simulink model "fft_filters"  (R2019b)
settings: Solver=FixedStepDiscrete  StartTime=0.0  StopTime=0.01  RelTol=1e-3
InitFcn:
  | initCallback
StopFcn:
  | stopCallback
undefined symbols (not defined in the file or in its folder): config, mp
libraries: hdlsllib x32, simulink x12, dsphdlxfrm x4, dspsigops x2
(part 1 of 2)
settings Model: DataTypeOverride=Off  SimulationMode=accelerator  Creator=Ross  LastModifiedBy=wickh
settings DataIOCC: ReturnWorkspaceOutputs=off
settings OptimizationCC: BlockReduction=off  ConditionallyExecuteInputs=off  DefaultParameterBehavior=Inlined
settings DebuggingCC: ReadBeforeWriteMsg=DisableAll  WriteAfterWriteMsg=DisableAll  WriteAfterReadMsg=DisableAll  AlgebraicLoopMsg=error  MultiTaskDSMMsg=none  SingleTaskRateTransMsg=error  PregeneratedLibrarySubsystemCodeDiagnostic=none  ArithmeticOperatorsInVariantConditions=warning
settings HardwareCC: ProdBitPerPointer=32  ProdBitPerSizeT=32  ProdBitPerPtrDiffT=32  ProdLargestAtomicFloat=None  ProdIntDivRoundTo=Undefined  ProdEndianess=Unspecified  ProdWordSize=32  ProdHWDeviceType=ASIC/FPGA->ASIC/FPGA  TargetBitPerPointer=64  TargetBitPerSizeT=64  TargetBitPerPtrDiffT=64  TargetLongLongMode=on  TargetIntDivRoundTo=Zero  TargetEndianess=LittleEndian  TargetWordSize=64  TargetHWDeviceType=Custom Processor->MATLAB Host Computer  ProdEqTarget=off
settings ModelReferenceCC: UpdateModelReferenceTargets=IfOutOfDate
settings SFSimCC: SFSimEcho=off  SimUseLocalCustomCode=off  CustomCodeUndefinedFunction=UseInterfaceOnly
settings RTWCC: RTWUseLocalCustomCode=off

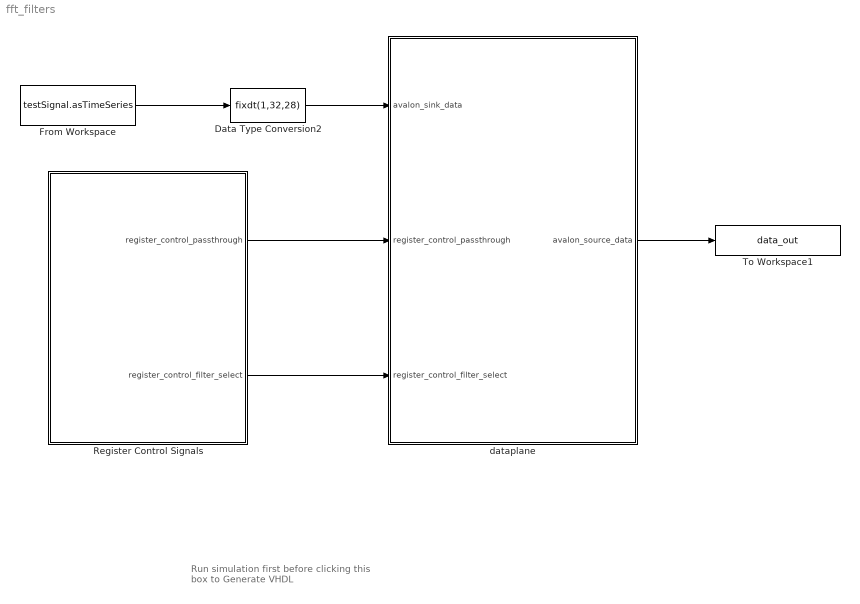
== system fft_filters ==
  note: Run simulation first
      | before clicking this box to
      | Generate VHDL
  Data Type Conversion2 : DataTypeConversion  OutDataTypeStr=fixdt(1,32,28)
  From Workspace : FromWorkspace  VariableName=testSignal.asTimeSeries  SampleTime=1 / config.system.sampleClockFrequency
  Register Control Signals : Subsystem
  To Workspace1 : ToWorkspace  VariableName=data_out  SaveFormat=Timeseries  SampleTime=-1
  dataplane : Subsystem  TreatAsAtomicUnit=on
  wires:
  dataplane/1("avalon_source_data ") -> To Workspace1/1
  Register Control Signals/1(register_control_passthrough) -> dataplane/2(register_control_passthrough)
  Register Control Signals/2(register_control_filter_select) -> dataplane/3(register_control_filter_select)
  From Workspace/1 -> Data Type Conversion2/1
  Data Type Conversion2/1 -> dataplane/1(avalon_sink_data)

== system fft_filters/Register Control Signals ==
  Data Type Conversion1 : DataTypeConversion  OutDataTypeStr=mp.register{2}.dataType  RndMeth=Nearest
  Data Type Conversion2 : DataTypeConversion  OutDataTypeStr=mp.register{1}.dataType  RndMeth=Nearest
  Time Series Signal from Workspace 1 : FromWorkspace  VariableName=mp.register{1}.timeseries  OutDataTypeStr=double  SampleTime=mp.Ts  OutputAfterFinalValue=Holding final value
  Time Series Signal from Workspace 2 : FromWorkspace  VariableName=mp.register{2}.timeseries  OutDataTypeStr=double  SampleTime=mp.Ts  OutputAfterFinalValue=Holding final value
  register_control_passthrough : Outport  VectorParamsAs1DForOutWhenUnconnected=off
  register_control_filter_select : Outport  Port=2  VectorParamsAs1DForOutWhenUnconnected=off
  wires:
  Time Series Signal from Workspace 1/1 -> Data Type Conversion2/1
  Time Series Signal from Workspace 2/1 -> Data Type Conversion1/1
  Data Type Conversion2/1 -> register_control_passthrough/1
  Data Type Conversion1/1 -> register_control_filter_select/1

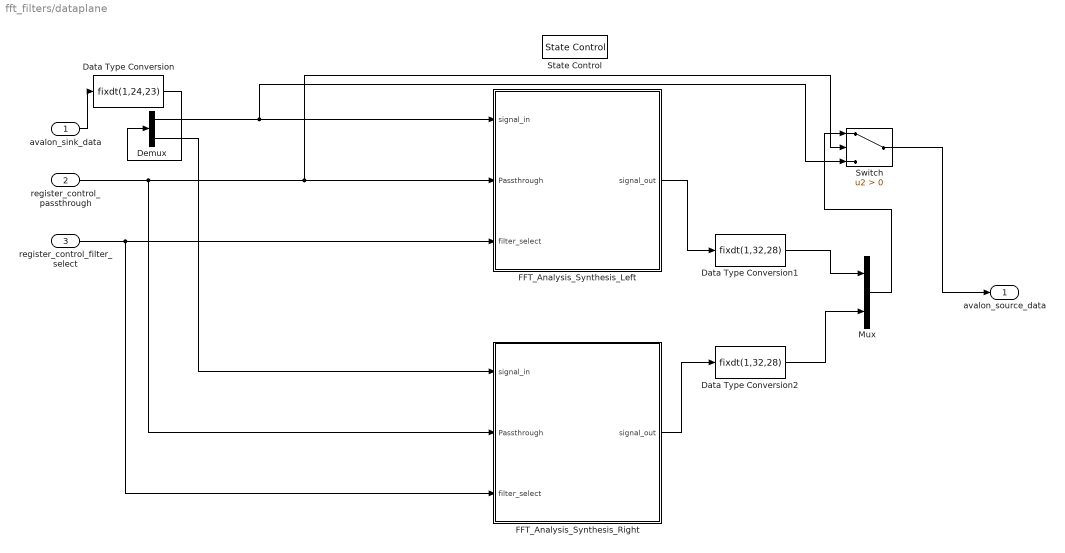
== system fft_filters/dataplane ==
  avalon_sink_data : Inport
  register_control_passthrough : Inport  Port=2
  register_control_filter_select : Inport  Port=3
  Data Type Conversion : DataTypeConversion  OutDataTypeStr=fixdt(1,24,23)
  Data Type Conversion1 : DataTypeConversion  OutDataTypeStr=fixdt(1,32,28)
  Data Type Conversion2 : DataTypeConversion  OutDataTypeStr=fixdt(1,32,28)
  Demux : Demux  Outputs=2
  FFT_Analysis_Synthesis_Left : Subsystem  TreatAsAtomicUnit=on
  FFT_Analysis_Synthesis_Right : Subsystem  TreatAsAtomicUnit=on
  Mux : Mux  Inputs=2
  State Control : StateControl  StateControl=Synchronous
  Switch : Switch  Criteria=u2 > Threshold
  "avalon_source_data " : Outport  InitialOutput=0  VectorParamsAs1DForOutWhenUnconnected=off
  wires:
  Demux/2 -> FFT_Analysis_Synthesis_Right/1(signal_in)
  FFT_Analysis_Synthesis_Right/1(signal_out) -> Data Type Conversion2/1
  avalon_sink_data/1 -> Data Type Conversion/1
  Demux/1 -> Switch/3, FFT_Analysis_Synthesis_Left/1(signal_in)
  FFT_Analysis_Synthesis_Left/1(signal_out) -> Data Type Conversion1/1
  register_control_passthrough/1 -> FFT_Analysis_Synthesis_Right/2(Passthrough), Switch/2, FFT_Analysis_Synthesis_Left/2(Passthrough)
  register_control_filter_select/1 -> FFT_Analysis_Synthesis_Left/3(filter_select), FFT_Analysis_Synthesis_Right/3(filter_select)
  Data Type Conversion/1 -> Demux/1
  Mux/1 -> Switch/1
  Data Type Conversion1/1 -> Mux/1
  Data Type Conversion2/1 -> Mux/2
  Switch/1 -> "avalon_source_data "/1

== system fft_filters/dataplane/FFT_Analysis_Synthesis_Left ==
  note: Gain to normalize
      | sinusoid amplitudes
  signal_in : Inport
  Passthrough : Inport  Port=2
  filter_select : Inport  Port=3
  Analysis : Subsystem
  Frequency_Domain_Processing : Subsystem
  Gain : Gain  OutDataTypeStr=Inherit: Same as input  ParamDataTypeStr=Inherit: Same as input
  Synthesis : Subsystem
  signal_out : Outport  VectorParamsAs1DForOutWhenUnconnected=off
  wires:
  signal_in/1 -> Analysis/1(Signal_in)
  Synthesis/1(synthesized_signal) -> Gain/1
  Analysis/1(FFT_data) -> Frequency_Domain_Processing/1(FFT_results)
  Analysis/2(FFT_valid) -> Frequency_Domain_Processing/2(valid_in)
  Analysis/3(FFT_frame_pulse) -> Frequency_Domain_Processing/3(frame_pulse_in)
  Frequency_Domain_Processing/1(modified_frequencies) -> Synthesis/1(modified_FFT_data)
  Frequency_Domain_Processing/2(valid_out) -> Synthesis/2(FFT_valid)
  Frequency_Domain_Processing/3(frame_pulse_out) -> Synthesis/3(FFT_frame_pulse)
  Analysis/4(passthrough) -> Frequency_Domain_Processing/4(passthrough)
  Passthrough/1 -> Analysis/2(Passthrough)
  Analysis/5(filter_select_out) -> Frequency_Domain_Processing/5(filter_select)
  filter_select/1 -> Analysis/3(filter_select)
  Gain/1 -> signal_out/1

== system fft_filters/dataplane/FFT_Analysis_Synthesis_Right ==
  note: Gain to normalize
      | sinusoid amplitudes
  signal_in : Inport
  Passthrough : Inport  Port=2
  filter_select : Inport  Port=3
  Analysis : Subsystem
  Frequency_Domain_Processing : Subsystem
  Gain : Gain  OutDataTypeStr=Inherit: Same as input  ParamDataTypeStr=Inherit: Same as input
  Synthesis : Subsystem
  signal_out : Outport  VectorParamsAs1DForOutWhenUnconnected=off
  wires:
  signal_in/1 -> Analysis/1(Signal_in)
  Synthesis/1(synthesized_signal) -> Gain/1
  Analysis/1(FFT_data) -> Frequency_Domain_Processing/1(FFT_results)
  Analysis/2(FFT_valid) -> Frequency_Domain_Processing/2(valid_in)
  Analysis/3(FFT_frame_pulse) -> Frequency_Domain_Processing/3(frame_pulse_in)
  Frequency_Domain_Processing/1(modified_frequencies) -> Synthesis/1(modified_FFT_data)
  Frequency_Domain_Processing/2(valid_out) -> Synthesis/2(FFT_valid)
  Frequency_Domain_Processing/3(frame_pulse_out) -> Synthesis/3(FFT_frame_pulse)
  Analysis/4(passthrough) -> Frequency_Domain_Processing/4(passthrough)
  Passthrough/1 -> Analysis/2(Passthrough)
  Analysis/5(filter_select_out) -> Frequency_Domain_Processing/5(filter_select)
  filter_select/1 -> Analysis/3(filter_select)
  Gain/1 -> signal_out/1

== system fft_filters/dataplane/FFT_Analysis_Synthesis_Left/Analysis ==
  note: The ready signal is ignored by design
      | since data won't be sent while FFT
      | engine is busy.
  Signal_in : Inport
  Passthrough : Inport  Port=2
  filter_select : Inport  Port=3
  FFT : dsphdlxfrm/FFT HDL Optimized  FFTLength=mp.FFT_size  Architecture=Burst Radix 2  ComplexMultiplication=Use 4 multipliers and 2 adders  BitReversedOutput=off  BitReversedInput=off  Normalize=off  SimulateUsing=Code generation  RoundingMethod=Floor  ResetInputPort=off  StartOutputPort=off  EndOutputPort=off
      settings: SourceProductName=DSP System Toolbox  SourceProductBaseCode=DS
  FFT Frame Buffering : Subsystem
  Terminator6 : Terminator
  FFT_data : Outport  VectorParamsAs1DForOutWhenUnconnected=off
  FFT_valid : Outport  Port=2  VectorParamsAs1DForOutWhenUnconnected=off
  FFT_frame_pulse : Outport  Port=3  VectorParamsAs1DForOutWhenUnconnected=off
  passthrough : Outport  Port=4
  filter_select_out : Outport  Port=5
  wires:
  FFT/3 -> Terminator6/1
  FFT Frame Buffering/3(FFT_Frame_Start_Pulse) -> FFT_frame_pulse/1
  Signal_in/1 -> FFT Frame Buffering/1(Sample_Data_in)
  FFT Frame Buffering/2(Valid_to_FFT) -> FFT/2
  FFT Frame Buffering/1(Data_to_FFT) -> FFT/1
  FFT/1 -> FFT_data/1
  FFT/2 -> FFT_valid/1
  FFT Frame Buffering/4(passthrough) -> passthrough/1
  Passthrough/1 -> FFT Frame Buffering/2(passthrough_in)
  filter_select/1 -> FFT Frame Buffering/3(filter_select)
  FFT Frame Buffering/5(filter_select_out) -> filter_select_out/1

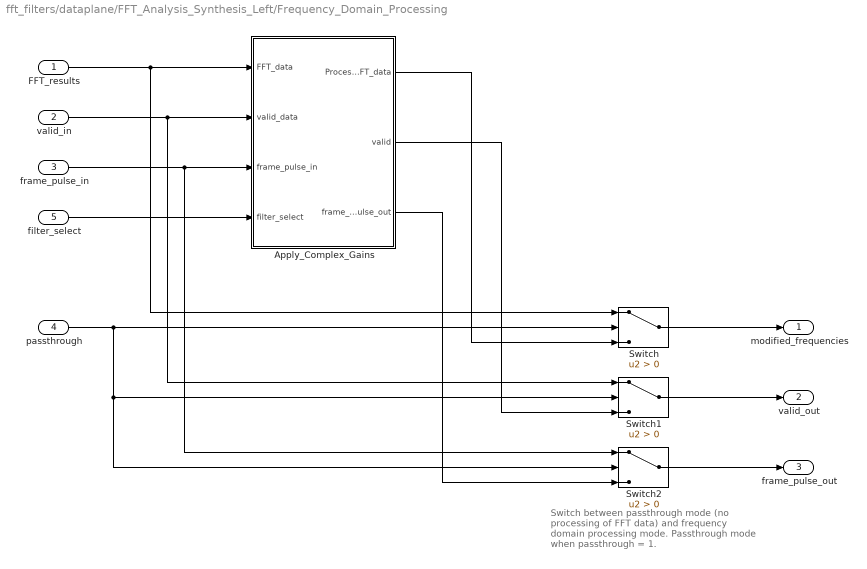
== system fft_filters/dataplane/FFT_Analysis_Synthesis_Left/Frequency_Domain_Processing ==
  note: Switch between passthrough mode
      | (no processing of FFT data)
      | and frequency domain processing mode.
      | Passthrough mode when passthrough = 1.
  FFT_results : Inport
  valid_in : Inport  Port=2
  frame_pulse_in : Inport  Port=3
  passthrough : Inport  Port=4
  filter_select : Inport  Port=5
  Apply_Complex_Gains : Subsystem
  Switch : Switch  Criteria=u2 > Threshold
  Switch1 : Switch  Criteria=u2 > Threshold
  Switch2 : Switch  Criteria=u2 > Threshold
  modified_frequencies : Outport  VectorParamsAs1DForOutWhenUnconnected=off
  valid_out : Outport  Port=2  VectorParamsAs1DForOutWhenUnconnected=off
  frame_pulse_out : Outport  Port=3
  wires:
  FFT_results/1 -> Apply_Complex_Gains/1(FFT_data), Switch/1
  valid_in/1 -> Apply_Complex_Gains/2(valid_data), Switch1/1
  Apply_Complex_Gains/1(Processed_FFT_data) -> Switch/3
  Apply_Complex_Gains/2(valid) -> Switch1/3
  frame_pulse_in/1 -> Apply_Complex_Gains/3(frame_pulse_in), Switch2/1
  passthrough/1 -> Switch2/2, Switch1/2, Switch/2
  Switch/1 -> modified_frequencies/1
  Apply_Complex_Gains/3(frame_pulse_out) -> Switch2/3
  Switch1/1 -> valid_out/1
  Switch2/1 -> frame_pulse_out/1
  filter_select/1 -> Apply_Complex_Gains/4(filter_select)

== system fft_filters/dataplane/FFT_Analysis_Synthesis_Left/Synthesis ==
  note: Making the assumption here
      | that the frequency domain processing
      | preserved the complex conjugate pairs
      | so that the output is real.
  modified_FFT_data : Inport
  FFT_valid : Inport  Port=2
  FFT_frame_pulse : Inport  Port=3
  Data Type Conversion1 : DataTypeConversion  OutDataTypeStr=fixdt(1,mp.W_bits,mp.F_bits)
  Get_Real : ComplexToRealImag
  Overlap_and_Add : Subsystem
  Terminator8 : Terminator
  Terminator9 : Terminator
  iFFT : dsphdlxfrm/IFFT HDL Optimized  FFTLength=mp.FFT_size  Architecture=Burst Radix 2  ComplexMultiplication=Use 4 multipliers and 2 adders  BitReversedOutput=off  BitReversedInput=off  Normalize=on  SimulateUsing=Code generation  RoundingMethod=Floor  ResetInputPort=off  StartOutputPort=off  EndOutputPort=off
      settings: SourceProductName=DSP System Toolbox  SourceProductBaseCode=DS
  synthesized_signal : Outport  VectorParamsAs1DForOutWhenUnconnected=off
  wires:
  iFFT/3 -> Terminator8/1
  iFFT/2 -> Overlap_and_Add/2(iFFT_Valid)
  Get_Real/1 -> Overlap_and_Add/1(IFFT_Data)
  modified_FFT_data/1 -> iFFT/1
  Data Type Conversion1/1 -> synthesized_signal/1
  iFFT/1 -> Get_Real/1
  Get_Real/2 -> Terminator9/1
  FFT_valid/1 -> iFFT/2
  FFT_frame_pulse/1 -> Overlap_and_Add/3(FFT_Frame_Pulse)
  Overlap_and_Add/1(signal_out) -> Data Type Conversion1/1

== system fft_filters/dataplane/FFT_Analysis_Synthesis_Right/Analysis ==
  note: The ready signal is ignored by design
      | since data won't be sent while FFT
      | engine is busy.
  Signal_in : Inport
  Passthrough : Inport  Port=2
  filter_select : Inport  Port=3
  FFT : dsphdlxfrm/FFT HDL Optimized  FFTLength=mp.FFT_size  Architecture=Burst Radix 2  ComplexMultiplication=Use 4 multipliers and 2 adders  BitReversedOutput=off  BitReversedInput=off  Normalize=off  SimulateUsing=Code generation  RoundingMethod=Floor  ResetInputPort=off  StartOutputPort=off  EndOutputPort=off
      settings: SourceProductName=DSP System Toolbox  SourceProductBaseCode=DS
  FFT Frame Buffering : Subsystem
  Terminator6 : Terminator
  FFT_data : Outport  VectorParamsAs1DForOutWhenUnconnected=off
  FFT_valid : Outport  Port=2  VectorParamsAs1DForOutWhenUnconnected=off
  FFT_frame_pulse : Outport  Port=3  VectorParamsAs1DForOutWhenUnconnected=off
  passthrough : Outport  Port=4
  filter_select_out : Outport  Port=5
  wires:
  FFT/3 -> Terminator6/1
  FFT Frame Buffering/3(FFT_Frame_Start_Pulse) -> FFT_frame_pulse/1
  Signal_in/1 -> FFT Frame Buffering/1(Sample_Data_in)
  FFT Frame Buffering/2(Valid_to_FFT) -> FFT/2
  FFT Frame Buffering/1(Data_to_FFT) -> FFT/1
  FFT/1 -> FFT_data/1
  FFT/2 -> FFT_valid/1
  FFT Frame Buffering/4(passthrough) -> passthrough/1
  Passthrough/1 -> FFT Frame Buffering/2(passthrough_in)
  filter_select/1 -> FFT Frame Buffering/3(filter_select)
  FFT Frame Buffering/5(filter_select_out) -> filter_select_out/1

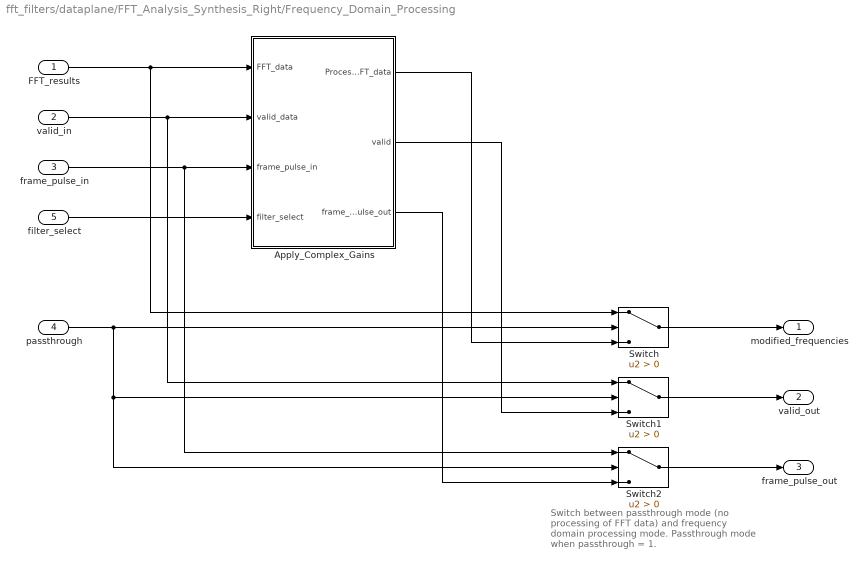
== system fft_filters/dataplane/FFT_Analysis_Synthesis_Right/Frequency_Domain_Processing ==
  note: Switch between passthrough mode
      | (no processing of FFT data)
      | and frequency domain processing mode.
      | Passthrough mode when passthrough = 1.
  FFT_results : Inport
  valid_in : Inport  Port=2
  frame_pulse_in : Inport  Port=3
  passthrough : Inport  Port=4
  filter_select : Inport  Port=5
  Apply_Complex_Gains : Subsystem
  Switch : Switch  Criteria=u2 > Threshold
  Switch1 : Switch  Criteria=u2 > Threshold
  Switch2 : Switch  Criteria=u2 > Threshold
  modified_frequencies : Outport  VectorParamsAs1DForOutWhenUnconnected=off
  valid_out : Outport  Port=2  VectorParamsAs1DForOutWhenUnconnected=off
  frame_pulse_out : Outport  Port=3
  wires:
  FFT_results/1 -> Apply_Complex_Gains/1(FFT_data), Switch/1
  valid_in/1 -> Apply_Complex_Gains/2(valid_data), Switch1/1
  Apply_Complex_Gains/1(Processed_FFT_data) -> Switch/3
  Apply_Complex_Gains/2(valid) -> Switch1/3
  frame_pulse_in/1 -> Apply_Complex_Gains/3(frame_pulse_in), Switch2/1
  passthrough/1 -> Switch2/2, Switch1/2, Switch/2
  Switch/1 -> modified_frequencies/1
  Apply_Complex_Gains/3(frame_pulse_out) -> Switch2/3
  Switch1/1 -> valid_out/1
  Switch2/1 -> frame_pulse_out/1
  filter_select/1 -> Apply_Complex_Gains/4(filter_select)

== system fft_filters/dataplane/FFT_Analysis_Synthesis_Right/Synthesis ==
  note: Making the assumption here
      | that the frequency domain processing
      | preserved the complex conjugate pairs
      | so that the output is real.
  modified_FFT_data : Inport
  FFT_valid : Inport  Port=2
  FFT_frame_pulse : Inport  Port=3
  Data Type Conversion1 : DataTypeConversion  OutDataTypeStr=fixdt(1,mp.W_bits,mp.F_bits)
  Get_Real : ComplexToRealImag
  Overlap_and_Add : Subsystem
  Terminator8 : Terminator
  Terminator9 : Terminator
  iFFT : dsphdlxfrm/IFFT HDL Optimized  FFTLength=mp.FFT_size  Architecture=Burst Radix 2  ComplexMultiplication=Use 4 multipliers and 2 adders  BitReversedOutput=off  BitReversedInput=off  Normalize=on  SimulateUsing=Code generation  RoundingMethod=Floor  ResetInputPort=off  StartOutputPort=off  EndOutputPort=off
      settings: SourceProductName=DSP System Toolbox  SourceProductBaseCode=DS
  synthesized_signal : Outport  VectorParamsAs1DForOutWhenUnconnected=off
  wires:
  iFFT/3 -> Terminator8/1
  iFFT/2 -> Overlap_and_Add/2(iFFT_Valid)
  Get_Real/1 -> Overlap_and_Add/1(IFFT_Data)
  modified_FFT_data/1 -> iFFT/1
  Data Type Conversion1/1 -> synthesized_signal/1
  iFFT/1 -> Get_Real/1
  Get_Real/2 -> Terminator9/1
  FFT_valid/1 -> iFFT/2
  FFT_frame_pulse/1 -> Overlap_and_Add/3(FFT_Frame_Pulse)
  Overlap_and_Add/1(signal_out) -> Data Type Conversion1/1

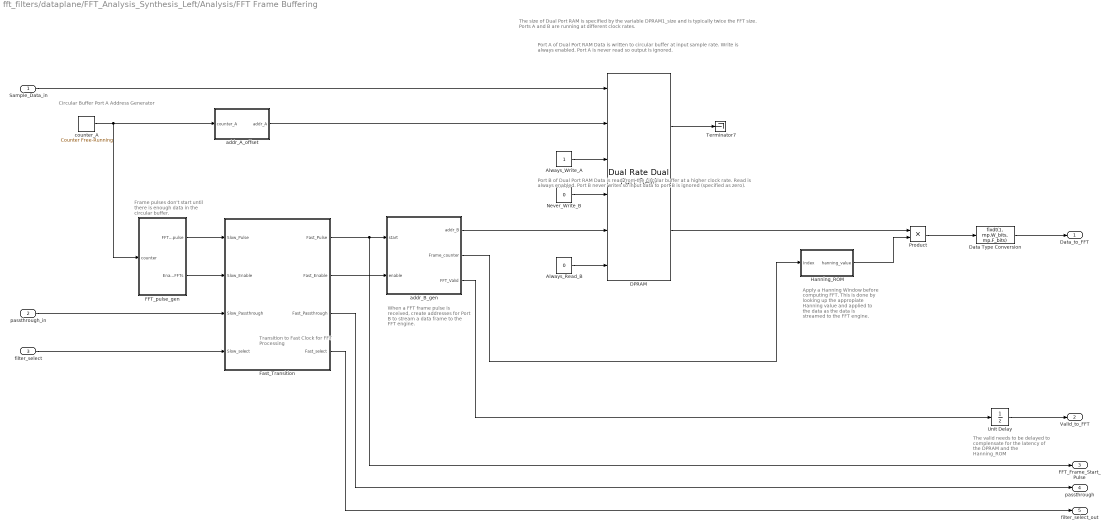
== system fft_filters/dataplane/FFT_Analysis_Synthesis_Left/Analysis/FFT Frame Buffering ==
  note: The valid needs to be delayed
      | to complensate for the latency
      | of the DPRAM and the
      | Hanning_ROM
  note: When a FFT frame pulse
      | is received, create addresses for
      | Port B to stream a data frame
      | to the FFT engine.
  note: Apply a Hanning Window
      | before computing FFT.  This
      | is done by looking up the
      | appropiate Hanning value
      | and applied to the data as the
      | data is streamed to the
      | FFT engine.
  note: Frame pulses don't start
      | until there is enough data
      | in the circular buffer.
  note: The size of Dual Port RAM is specified by the variable DPRAM1_size
      | and is typically twice the FFT size.  Ports A and B are running at different clock rates.
  note: Circular Buffer
      | Port A Address Generator
  note: Port A of Dual Port RAM
      |
      | Data is written to circular buffer at input sample rate.
      | Write is always enabled.  Port A is never read so output is ignored.
  note: Transition to
      | Fast Clock
      | for FFT Processing
  note: Port B of Dual Port RAM
      |
      | Data is read from the circular buffer at a higher clock rate.
      | Read is always enabled.  Port B never writes so input data to port B
      | is ignored (specified as zero).
  Sample_Data_in : Inport
  passthrough_in : Inport  Port=2
  filter_select : Inport  Port=3
  Always_Read_B : Constant  Value=0  OutDataTypeStr=boolean  SampleTime=mp.Ts/mp.SysRate_Upsample_Factor
  Always_Write_A : Constant  OutDataTypeStr=boolean  SampleTime=mp.Ts
  DPRAM : hdlsllib/HDL RAMs/Dual Rate Dual Port RAM  ram_size=mp.DPRAM1_address_size
      settings: SourceProductName=Simulink  SourceProductBaseCode=SL
  Data Type Conversion : DataTypeConversion  OutDataTypeStr=fixdt(1, mp.W_bits, mp.F_bits)
  FFT_pulse_gen : Subsystem
  Fast_Transition : Subsystem
  Hanning_ROM : Subsystem
  Never_Write_B : Constant  Value=0  OutDataTypeStr=fixdt(1,24,23)  SampleTime=mp.Ts/mp.SysRate_Upsample_Factor
  Product : Product
  Terminator7 : Terminator
  Unit Delay : UnitDelay  SampleTime=-1  HasFrameUpgradeWarning=on
  addr_A_offset : Subsystem
  addr_B_gen : Subsystem
  counter_A : simulink/Sources/Counter Free-Running  NumBits=mp.DPRAM1_address_size  tsamp=mp.Ts
  Data_to_FFT : Outport  VectorParamsAs1DForOutWhenUnconnected=off
  Valid_to_FFT : Outport  Port=2  VectorParamsAs1DForOutWhenUnconnected=off
  FFT_Frame_Start_Pulse : Outport  Port=3  VectorParamsAs1DForOutWhenUnconnected=off
  passthrough : Outport  Port=4
  filter_select_out : Outport  Port=5
  wires:
  Always_Write_A/1 -> DPRAM/3
  Never_Write_B/1 -> DPRAM/4
  Always_Read_B/1 -> DPRAM/6
  DPRAM/1 -> Terminator7/1
  addr_B_gen/3(FFT_Valid) -> Unit Delay/1
  addr_B_gen/1(addr_B) -> DPRAM/5
  counter_A/1 -> addr_A_offset/1(counter_A), FFT_pulse_gen/1(counter)
  Sample_Data_in/1 -> DPRAM/1
  addr_A_offset/1(addr_A) -> DPRAM/2
  addr_B_gen/2(Frame_counter) -> Hanning_ROM/1(Index)
  Product/1 -> Data Type Conversion/1
  DPRAM/2 -> Product/1
  Hanning_ROM/1(hanning_value) -> Product/2
  Data Type Conversion/1 -> Data_to_FFT/1
  Fast_Transition/1(Fast_Pulse) -> FFT_Frame_Start_Pulse/1, addr_B_gen/1(start)
  FFT_pulse_gen/1(FFT_start_pulse) -> Fast_Transition/1(Slow_Pulse)
  FFT_pulse_gen/2(Enable_FFTs) -> Fast_Transition/2(Slow_Enable)
  Fast_Transition/2(Fast_Enable) -> addr_B_gen/2(enable)
  Unit Delay/1 -> Valid_to_FFT/1
  passthrough_in/1 -> Fast_Transition/3(Slow_Passthrough)
  Fast_Transition/3(Fast_Passthrough) -> passthrough/1
  filter_select/1 -> Fast_Transition/4(Slow_select)
  Fast_Transition/4(Fast_select) -> filter_select_out/1

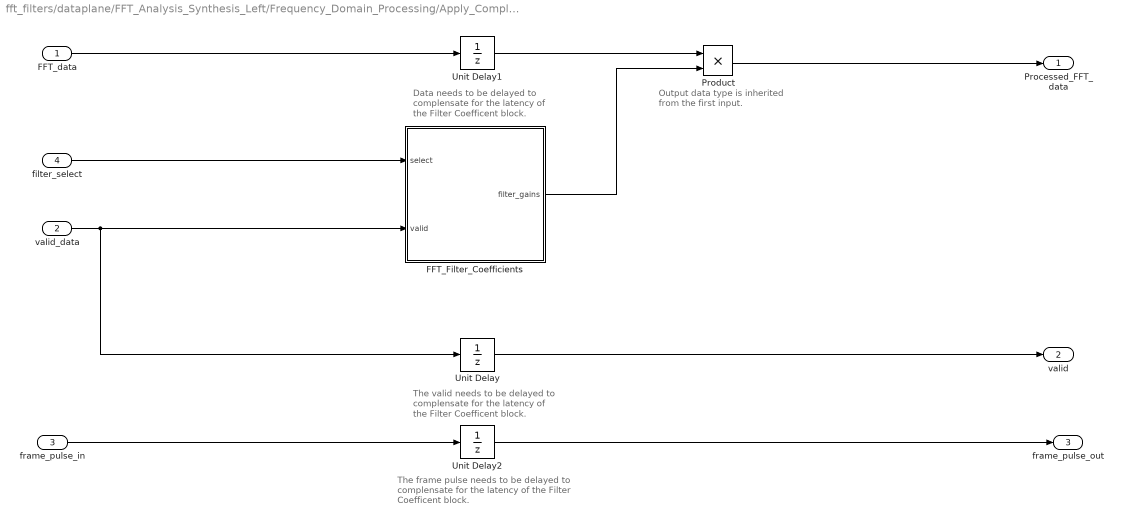
== system fft_filters/dataplane/FFT_Analysis_Synthesis_Left/Frequency_Domain_Processing/Apply_Complex_Gains ==
  note: Output data type is inherited
      | from the first input.
  note: The frame pulse needs to be delayed
      | to complensate for the latency
      | of the Filter Coefficent block.
  note: The valid needs to be delayed
      | to complensate for the latency
      | of the Filter Coefficent block.
  note: Data needs to be delayed
      | to complensate for the latency
      | of the Filter Coefficent block.
  FFT_data : Inport
  valid_data : Inport  Port=2
  frame_pulse_in : Inport  Port=3
  filter_select : Inport  Port=4
  FFT_Filter_Coefficients : Subsystem
  Product : Product  OutDataTypeStr=Inherit: Same as first input
  Unit Delay : UnitDelay  SampleTime=-1  HasFrameUpgradeWarning=on
  Unit Delay1 : UnitDelay  SampleTime=-1  HasFrameUpgradeWarning=on
  Unit Delay2 : UnitDelay  SampleTime=-1  HasFrameUpgradeWarning=on
  Processed_FFT_data : Outport
  valid : Outport  Port=2
  frame_pulse_out : Outport  Port=3
  wires:
  valid_data/1 -> Unit Delay/1, FFT_Filter_Coefficients/2(valid)
  FFT_data/1 -> Unit Delay1/1
  frame_pulse_in/1 -> Unit Delay2/1
  Unit Delay2/1 -> frame_pulse_out/1
  filter_select/1 -> FFT_Filter_Coefficients/1(select)
  FFT_Filter_Coefficients/1(filter_gains) -> Product/2
  Product/1 -> Processed_FFT_data/1
  Unit Delay/1 -> valid/1
  Unit Delay1/1 -> Product/1

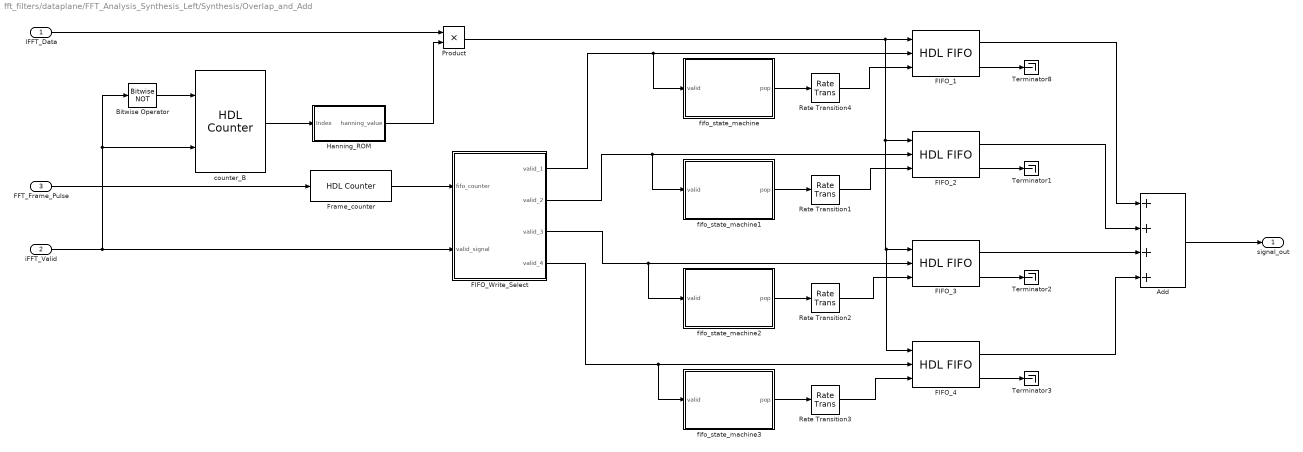
== system fft_filters/dataplane/FFT_Analysis_Synthesis_Left/Synthesis/Overlap_and_Add ==
  IFFT_Data : Inport
  iFFT_Valid : Inport  Port=2
  FFT_Frame_Pulse : Inport  Port=3
  Add : Sum  Inputs=4
  Bitwise Operator : simulink/Logic and Bit Operations/Bitwise Operator  logicop=NOT  UseBitMask=off  BitMask=bin2dec('11011001')  BitMaskRealWorld=Stored Integer
  FIFO_{1..4} (4 alike) : hdlsllib/HDL RAMs/HDL FIFO  fifo_size=mp.FFT_size  mode=Classic  ratio=mp.SysRate_Upsample_Factor  push_msg=Warning  pop_msg=Warning  show_empty=off  show_full=on  show_num=off  LabelModeActiveChoice_Mode=Classic
      settings: SourceProductName=Simulink  SourceProductBaseCode=SL
  FIFO_Write_Select : MATLAB Function  TreatAsAtomicUnit=on
  Frame_counter : hdlsllib/Sources/HDL Counter  CountType=Free running  CountInit=2  CountStep=1  CountMax=1024  CountFromType=Initial value  CountFrom=2  CountResetPort=off  CountLoadPort=off  CountEnbPort=on  CountDirPort=off  CountDataType=Unsigned  CountWordLen=2  CountFracLen=0  CountSampTime=1
      settings: SourceProductName=Simulink
  Hanning_ROM : Subsystem
  Product : Product  OutDataTypeStr=Inherit: Same as first input
  Rate Transition{1..4} (4 alike) : RateTransition  OutPortSampleTimeOpt=Multiple of input port sample time  OutPortSampleTimeMultiple=mp.SysRate_Upsample_Factor
  Terminator{1..3,8} (4 alike) : Terminator
  counter_B : hdlsllib/Sources/HDL Counter  CountType=Count limited  CountInit=0  CountStep=1  CountMax=mp.FFT_size  CountFromType=Initial value  CountFrom=0  CountResetPort=on  CountLoadPort=off  CountEnbPort=on  CountDirPort=off  CountDataType=Unsigned  CountWordLen=mp.DPRAM1_address_size  CountFracLen=0  CountSampTime=1
      settings: SourceProductName=Simulink
  fifo_state_machine : MATLAB Function  TreatAsAtomicUnit=on
  fifo_state_machine1 : MATLAB Function  TreatAsAtomicUnit=on
  fifo_state_machine2 : MATLAB Function  TreatAsAtomicUnit=on
  fifo_state_machine3 : MATLAB Function  TreatAsAtomicUnit=on
  signal_out : Outport  VectorParamsAs1DForOutWhenUnconnected=off
  wires:
  FIFO_1/1 -> Add/1
  FIFO_3/1 -> Add/3
  FFT_Frame_Pulse/1 -> Frame_counter/1
  FIFO_2/1 -> Add/2
  FIFO_Write_Select/3(valid_3) -> fifo_state_machine2/1(valid), FIFO_3/2
  FIFO_Write_Select/4(valid_4) -> fifo_state_machine3/1(valid), FIFO_4/2
  FIFO_4/1 -> Add/4
  FIFO_Write_Select/1(valid_1) -> fifo_state_machine/1(valid), FIFO_1/2
  FIFO_Write_Select/2(valid_2) -> fifo_state_machine1/1(valid), FIFO_2/2
  Add/1 -> signal_out/1
  Frame_counter/1 -> FIFO_Write_Select/1(fifo_counter)
  FIFO_4/2 -> Terminator3/1
  FIFO_2/2 -> Terminator1/1
  FIFO_3/2 -> Terminator2/1
  Bitwise Operator/1 -> counter_B/1
  iFFT_Valid/1 -> counter_B/2, Bitwise Operator/1, FIFO_Write_Select/2(valid_signal)
  IFFT_Data/1 -> Product/1
  Hanning_ROM/1(hanning_value) -> Product/2
  counter_B/1 -> Hanning_ROM/1(Index)
  fifo_state_machine/1(pop) -> Rate Transition4/1
  Rate Transition4/1 -> FIFO_1/3
  FIFO_1/2 -> Terminator8/1
  fifo_state_machine1/1(pop) -> Rate Transition1/1
  Rate Transition1/1 -> FIFO_2/3
  fifo_state_machine2/1(pop) -> Rate Transition2/1
  Rate Transition2/1 -> FIFO_3/3
  fifo_state_machine3/1(pop) -> Rate Transition3/1
  Rate Transition3/1 -> FIFO_4/3
  Product/1 -> FIFO_4/1, FIFO_3/1, FIFO_2/1, FIFO_1/1

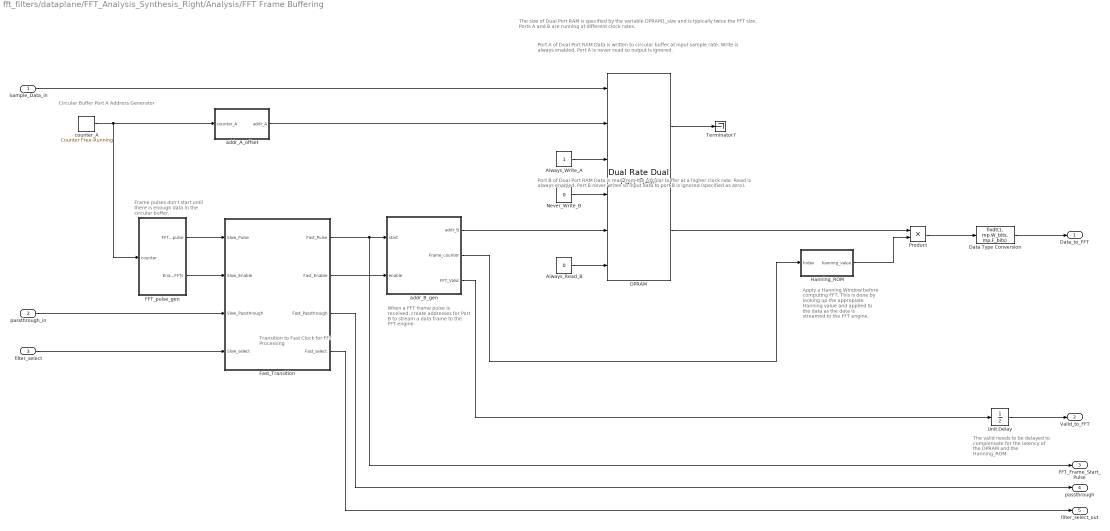
== system fft_filters/dataplane/FFT_Analysis_Synthesis_Right/Analysis/FFT Frame Buffering ==
  note: The valid needs to be delayed
      | to complensate for the latency
      | of the DPRAM and the
      | Hanning_ROM
  note: When a FFT frame pulse
      | is received, create addresses for
      | Port B to stream a data frame
      | to the FFT engine.
  note: Apply a Hanning Window
      | before computing FFT.  This
      | is done by looking up the
      | appropiate Hanning value
      | and applied to the data as the
      | data is streamed to the
      | FFT engine.
  note: Frame pulses don't start
      | until there is enough data
      | in the circular buffer.
  note: The size of Dual Port RAM is specified by the variable DPRAM1_size
      | and is typically twice the FFT size.  Ports A and B are running at different clock rates.
  note: Circular Buffer
      | Port A Address Generator
  note: Port A of Dual Port RAM
      |
      | Data is written to circular buffer at input sample rate.
      | Write is always enabled.  Port A is never read so output is ignored.
  note: Transition to
      | Fast Clock
      | for FFT Processing
  note: Port B of Dual Port RAM
      |
      | Data is read from the circular buffer at a higher clock rate.
      | Read is always enabled.  Port B never writes so input data to port B
      | is ignored (specified as zero).
  Sample_Data_in : Inport
  passthrough_in : Inport  Port=2
  filter_select : Inport  Port=3
  Always_Read_B : Constant  Value=0  OutDataTypeStr=boolean  SampleTime=mp.Ts/mp.SysRate_Upsample_Factor
  Always_Write_A : Constant  OutDataTypeStr=boolean  SampleTime=mp.Ts
  DPRAM : hdlsllib/HDL RAMs/Dual Rate Dual Port RAM  ram_size=mp.DPRAM1_address_size
      settings: SourceProductName=Simulink  SourceProductBaseCode=SL
  Data Type Conversion : DataTypeConversion  OutDataTypeStr=fixdt(1, mp.W_bits, mp.F_bits)
  FFT_pulse_gen : Subsystem
  Fast_Transition : Subsystem
  Hanning_ROM : Subsystem
  Never_Write_B : Constant  Value=0  OutDataTypeStr=fixdt(1,24,23)  SampleTime=mp.Ts/mp.SysRate_Upsample_Factor
  Product : Product
  Terminator7 : Terminator
  Unit Delay : UnitDelay  SampleTime=-1  HasFrameUpgradeWarning=on
  addr_A_offset : Subsystem
  addr_B_gen : Subsystem
  counter_A : simulink/Sources/Counter Free-Running  NumBits=mp.DPRAM1_address_size  tsamp=mp.Ts
  Data_to_FFT : Outport  VectorParamsAs1DForOutWhenUnconnected=off
  Valid_to_FFT : Outport  Port=2  VectorParamsAs1DForOutWhenUnconnected=off
  FFT_Frame_Start_Pulse : Outport  Port=3  VectorParamsAs1DForOutWhenUnconnected=off
  passthrough : Outport  Port=4
  filter_select_out : Outport  Port=5
  wires:
  Always_Write_A/1 -> DPRAM/3
  Never_Write_B/1 -> DPRAM/4
  Always_Read_B/1 -> DPRAM/6
  DPRAM/1 -> Terminator7/1
  addr_B_gen/3(FFT_Valid) -> Unit Delay/1
  addr_B_gen/1(addr_B) -> DPRAM/5
  counter_A/1 -> addr_A_offset/1(counter_A), FFT_pulse_gen/1(counter)
  Sample_Data_in/1 -> DPRAM/1
  addr_A_offset/1(addr_A) -> DPRAM/2
  addr_B_gen/2(Frame_counter) -> Hanning_ROM/1(Index)
  Product/1 -> Data Type Conversion/1
  DPRAM/2 -> Product/1
  Hanning_ROM/1(hanning_value) -> Product/2
  Data Type Conversion/1 -> Data_to_FFT/1
  Fast_Transition/1(Fast_Pulse) -> FFT_Frame_Start_Pulse/1, addr_B_gen/1(start)
  FFT_pulse_gen/1(FFT_start_pulse) -> Fast_Transition/1(Slow_Pulse)
  FFT_pulse_gen/2(Enable_FFTs) -> Fast_Transition/2(Slow_Enable)
  Fast_Transition/2(Fast_Enable) -> addr_B_gen/2(enable)
  Unit Delay/1 -> Valid_to_FFT/1
  passthrough_in/1 -> Fast_Transition/3(Slow_Passthrough)
  Fast_Transition/3(Fast_Passthrough) -> passthrough/1
  filter_select/1 -> Fast_Transition/4(Slow_select)
  Fast_Transition/4(Fast_select) -> filter_select_out/1

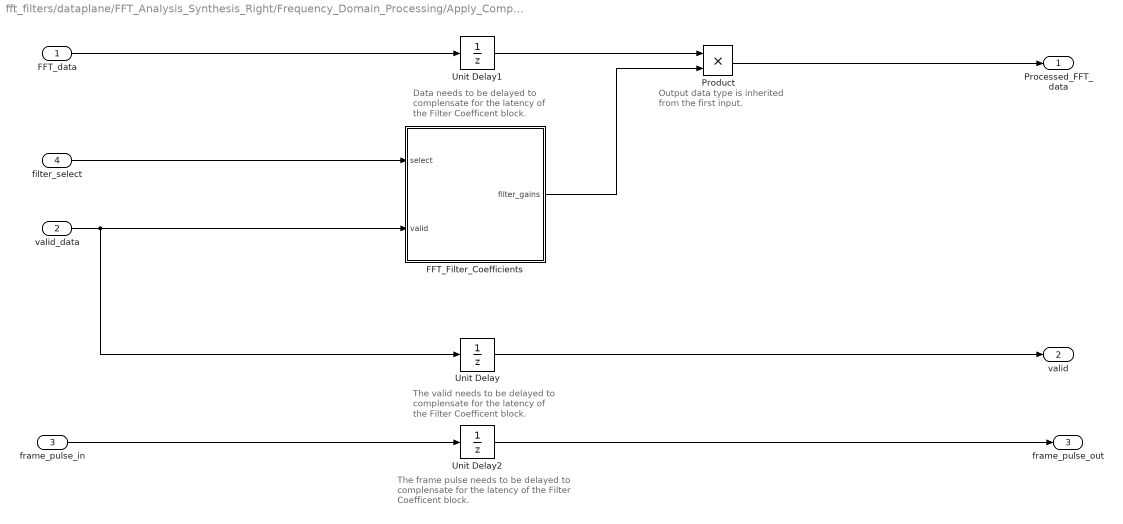
== system fft_filters/dataplane/FFT_Analysis_Synthesis_Right/Frequency_Domain_Processing/Apply_Complex_Gains ==
  note: Output data type is inherited
      | from the first input.
  note: The frame pulse needs to be delayed
      | to complensate for the latency
      | of the Filter Coefficent block.
  note: The valid needs to be delayed
      | to complensate for the latency
      | of the Filter Coefficent block.
  note: Data needs to be delayed
      | to complensate for the latency
      | of the Filter Coefficent block.
  FFT_data : Inport
  valid_data : Inport  Port=2
  frame_pulse_in : Inport  Port=3
  filter_select : Inport  Port=4
  FFT_Filter_Coefficients : Subsystem
  Product : Product  OutDataTypeStr=Inherit: Same as first input
  Unit Delay : UnitDelay  SampleTime=-1  HasFrameUpgradeWarning=on
  Unit Delay1 : UnitDelay  SampleTime=-1  HasFrameUpgradeWarning=on
  Unit Delay2 : UnitDelay  SampleTime=-1  HasFrameUpgradeWarning=on
  Processed_FFT_data : Outport
  valid : Outport  Port=2
  frame_pulse_out : Outport  Port=3
  wires:
  valid_data/1 -> Unit Delay/1, FFT_Filter_Coefficients/2(valid)
  FFT_data/1 -> Unit Delay1/1
  frame_pulse_in/1 -> Unit Delay2/1
  Unit Delay2/1 -> frame_pulse_out/1
  filter_select/1 -> FFT_Filter_Coefficients/1(select)
  FFT_Filter_Coefficients/1(filter_gains) -> Product/2
  Product/1 -> Processed_FFT_data/1
  Unit Delay/1 -> valid/1
  Unit Delay1/1 -> Product/1

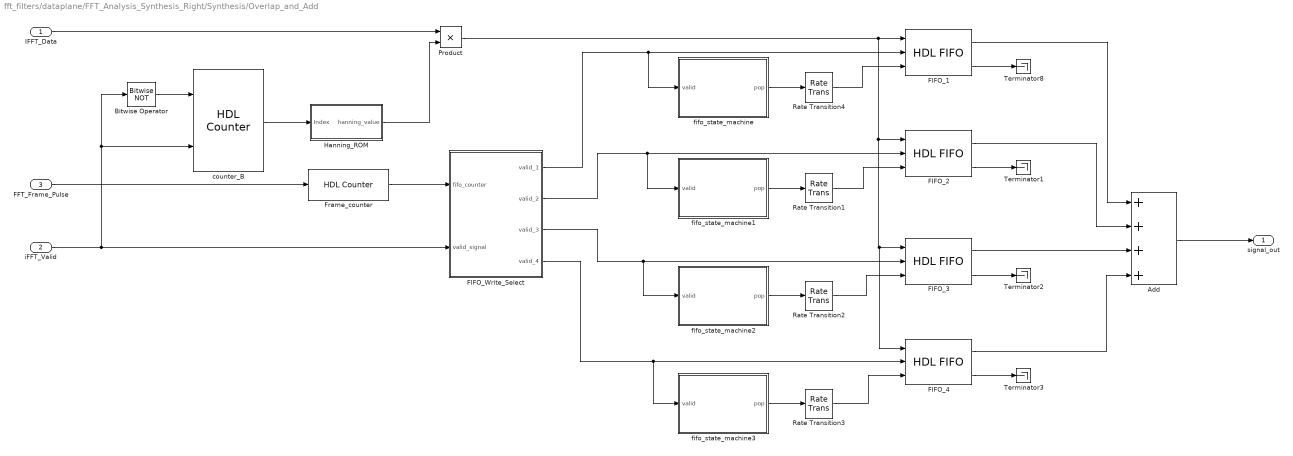
== system fft_filters/dataplane/FFT_Analysis_Synthesis_Right/Synthesis/Overlap_and_Add ==
  IFFT_Data : Inport
  iFFT_Valid : Inport  Port=2
  FFT_Frame_Pulse : Inport  Port=3
  Add : Sum  Inputs=4
  Bitwise Operator : simulink/Logic and Bit Operations/Bitwise Operator  logicop=NOT  UseBitMask=off  BitMask=bin2dec('11011001')  BitMaskRealWorld=Stored Integer
  FIFO_{1..4} (4 alike) : hdlsllib/HDL RAMs/HDL FIFO  fifo_size=mp.FFT_size  mode=Classic  ratio=mp.SysRate_Upsample_Factor  push_msg=Warning  pop_msg=Warning  show_empty=off  show_full=on  show_num=off  LabelModeActiveChoice_Mode=Classic
      settings: SourceProductName=Simulink  SourceProductBaseCode=SL
  FIFO_Write_Select : MATLAB Function  TreatAsAtomicUnit=on
  Frame_counter : hdlsllib/Sources/HDL Counter  CountType=Free running  CountInit=2  CountStep=1  CountMax=1024  CountFromType=Initial value  CountFrom=2  CountResetPort=off  CountLoadPort=off  CountEnbPort=on  CountDirPort=off  CountDataType=Unsigned  CountWordLen=2  CountFracLen=0  CountSampTime=1
      settings: SourceProductName=Simulink
  Hanning_ROM : Subsystem
  Product : Product  OutDataTypeStr=Inherit: Same as first input
  Rate Transition{1..4} (4 alike) : RateTransition  OutPortSampleTimeOpt=Multiple of input port sample time  OutPortSampleTimeMultiple=mp.SysRate_Upsample_Factor
  Terminator{1..3,8} (4 alike) : Terminator
  counter_B : hdlsllib/Sources/HDL Counter  CountType=Count limited  CountInit=0  CountStep=1  CountMax=mp.FFT_size  CountFromType=Initial value  CountFrom=0  CountResetPort=on  CountLoadPort=off  CountEnbPort=on  CountDirPort=off  CountDataType=Unsigned  CountWordLen=mp.DPRAM1_address_size  CountFracLen=0  CountSampTime=1
      settings: SourceProductName=Simulink
  fifo_state_machine : MATLAB Function  TreatAsAtomicUnit=on
  fifo_state_machine1 : MATLAB Function  TreatAsAtomicUnit=on
  fifo_state_machine2 : MATLAB Function  TreatAsAtomicUnit=on
  fifo_state_machine3 : MATLAB Function  TreatAsAtomicUnit=on
  signal_out : Outport  VectorParamsAs1DForOutWhenUnconnected=off
  wires:
  FIFO_1/1 -> Add/1
  FIFO_3/1 -> Add/3
  FFT_Frame_Pulse/1 -> Frame_counter/1
  FIFO_2/1 -> Add/2
  FIFO_Write_Select/3(valid_3) -> fifo_state_machine2/1(valid), FIFO_3/2
  FIFO_Write_Select/4(valid_4) -> fifo_state_machine3/1(valid), FIFO_4/2
  FIFO_4/1 -> Add/4
  FIFO_Write_Select/1(valid_1) -> fifo_state_machine/1(valid), FIFO_1/2
  FIFO_Write_Select/2(valid_2) -> fifo_state_machine1/1(valid), FIFO_2/2
  Add/1 -> signal_out/1
  Frame_counter/1 -> FIFO_Write_Select/1(fifo_counter)
  FIFO_4/2 -> Terminator3/1
  FIFO_2/2 -> Terminator1/1
  FIFO_3/2 -> Terminator2/1
  Bitwise Operator/1 -> counter_B/1
  iFFT_Valid/1 -> counter_B/2, Bitwise Operator/1, FIFO_Write_Select/2(valid_signal)
  IFFT_Data/1 -> Product/1
  Hanning_ROM/1(hanning_value) -> Product/2
  counter_B/1 -> Hanning_ROM/1(Index)
  fifo_state_machine/1(pop) -> Rate Transition4/1
  Rate Transition4/1 -> FIFO_1/3
  FIFO_1/2 -> Terminator8/1
  fifo_state_machine1/1(pop) -> Rate Transition1/1
  Rate Transition1/1 -> FIFO_2/3
  fifo_state_machine2/1(pop) -> Rate Transition2/1
  Rate Transition2/1 -> FIFO_3/3
  Rate Transition3/1 -> FIFO_4/3
  Product/1 -> FIFO_4/1, FIFO_3/1, FIFO_2/1, FIFO_1/1
  fifo_state_machine3/1(pop) -> Rate Transition3/1

== system fft_filters/dataplane/FFT_Analysis_Synthesis_Left/Analysis/FFT Frame Buffering/FFT_pulse_gen ==
  note: Don't send out FFT frame start pulses
      | until circular buffer has filled.
  counter : Inport
  FFT_Frame_Pulse_Gen : Subsystem
  Wait_for_data_to_start : Subsystem
  FFT_start_pulse : Outport  VectorParamsAs1DForOutWhenUnconnected=off
  Enable_FFTs : Outport  Port=2  VectorParamsAs1DForOutWhenUnconnected=off
  wires:
  counter/1 -> FFT_Frame_Pulse_Gen/1("counter_value ")
  Wait_for_data_to_start/1(FFT_Frame_Start) -> FFT_start_pulse/1
  Wait_for_data_to_start/2(Enable_FFT_Frames) -> Enable_FFTs/1
  FFT_Frame_Pulse_Gen/1(Frame_Pulse) -> Wait_for_data_to_start/1(Frame_Pulse)

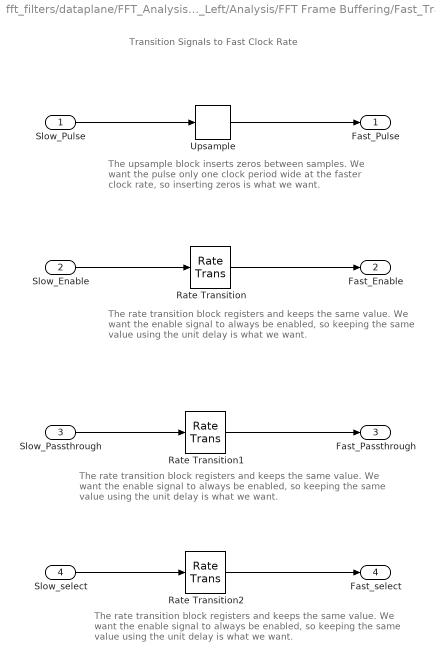
== system fft_filters/dataplane/FFT_Analysis_Synthesis_Left/Analysis/FFT Frame Buffering/Fast_Transition ==
  note: The upsample block inserts zeros between samples.
      | We want the pulse only one clock period wide at the
      | faster clock rate, so inserting zeros is what we want.
  note: Transition Signals to Fast Clock Rate
  note: The rate transition block registers and keeps the same
      | value.  We want the enable signal to always be enabled,
      | so keeping the same value using the unit delay is what we want.
  note: The rate transition block registers and keeps the same
      | value.  We want the enable signal to always be enabled,
      | so keeping the same value using the unit delay is what we want.
  note: The rate transition block registers and keeps the same
      | value.  We want the enable signal to always be enabled,
      | so keeping the same value using the unit delay is what we want.
  Slow_Pulse : Inport
  Slow_Enable : Inport  Port=2
  Slow_Passthrough : Inport  Port=3
  Slow_select : Inport  Port=4
  Rate Transition : RateTransition  OutPortSampleTimeOpt=Multiple of input port sample time  OutPortSampleTimeMultiple=1/mp.SysRate_Upsample_Factor
  Rate Transition1 : RateTransition  OutPortSampleTimeOpt=Multiple of input port sample time  OutPortSampleTimeMultiple=1/mp.SysRate_Upsample_Factor
  Rate Transition2 : RateTransition  InitialCondition=3  OutPortSampleTimeOpt=Multiple of input port sample time  OutPortSampleTimeMultiple=1/mp.SysRate_Upsample_Factor
  Upsample : dspsigops/Upsample  N=mp.SysRate_Upsample_Factor  phase=0  RateOptions=Allow multirate processing  ic=0  mode=Unused parameter value
  Fast_Pulse : Outport
  Fast_Enable : Outport  Port=2
  Fast_Passthrough : Outport  Port=3
  Fast_select : Outport  Port=4
  wires:
  Slow_Pulse/1 -> Upsample/1
  Rate Transition/1 -> Fast_Enable/1
  Slow_Enable/1 -> Rate Transition/1
  Upsample/1 -> Fast_Pulse/1
  Slow_Passthrough/1 -> Rate Transition1/1
  Rate Transition1/1 -> Fast_Passthrough/1
  Slow_select/1 -> Rate Transition2/1
  Rate Transition2/1 -> Fast_select/1

== system fft_filters/dataplane/FFT_Analysis_Synthesis_Left/Analysis/FFT Frame Buffering/Hanning_ROM ==
  Index : Inport
  Bit Slice : hdlsllib/Logic and Bit Operations/Bit Slice  lidx=log2(mp.FFT_size) - 1  ridx=0
      settings: SourceProductName=Simulink  SourceProductBaseCode=SL
  Lookup Table : Lookup_n-D  NumberOfTableDimensions=1  BreakpointsForDimension1=[0:mp.FFT_size-1]  IndexSearchMethod=Evenly spaced points  Table=hanning(mp.FFT_size)  InterpMethod=Flat  ExtrapMethod=Clip  DiagnosticForOutOfRangeInput=Warning  UseLastTableValue=on  OutDataTypeStr=fixdt(1,24,23)  RndMeth=Simplest  InputSameDT=on
  Unit Delay : UnitDelay  SampleTime=-1  HasFrameUpgradeWarning=on
  hanning_value : Outport  VectorParamsAs1DForOutWhenUnconnected=off
  wires:
  Unit Delay/1 -> hanning_value/1
  Index/1 -> Bit Slice/1
  Lookup Table/1 -> Unit Delay/1
  Bit Slice/1 -> Lookup Table/1

== system fft_filters/dataplane/FFT_Analysis_Synthesis_Left/Analysis/FFT Frame Buffering/addr_A_offset ==
  note: Adding 1 to counter since the read pointer (addr_B) can catch the write pointer (addr_A)
      | if SysRate_Upsample_Factor is large enough and Simulink will throw an error.
      | It would be nice if the HDL Coder allowed a read-before-write option when
      | the addresses are identical, which some memories support.
  counter_A : Inport
  Add : Sum  OutDataTypeStr=fixdt(0,mp.DPRAM1_address_size,0)
  write_offset : Constant  OutDataTypeStr=fixdt(0,mp.DPRAM1_address_size,0)  SampleTime=mp.Ts
  addr_A : Outport  VectorParamsAs1DForOutWhenUnconnected=off
  wires:
  write_offset/1 -> Add/2
  Add/1 -> addr_A/1
  counter_A/1 -> Add/1

== system fft_filters/dataplane/FFT_Analysis_Synthesis_Left/Analysis/FFT Frame Buffering/addr_B_gen ==
  note: Counter values [0 FFT_size-1] that
      | is used to lookup the window values
      | being applied.
  note: Valid data is being streamed to the FFT Engine.
  note: Enable signal that indicates
      | there is data in the buffer
      | and FFTs can start.
  note: The start pulse sets the starting count to Start_Address
      |  and the counter counts from Start_Address to Start_Address + FFT_size - 1
      | which is the address sent to Port B of the dual port memory.
  start : Inport
  enable : Inport  Port=2
  Logical Operator1 : Logic  AllPortsSameDT=off  OutDataTypeStr=boolean
  addr_B_gen_enable : Subsystem
  counter_B : hdlsllib/Sources/HDL Counter  CountType=Free running  CountInit=mp.DPRAM1_size-10  CountStep=1  CountMax=1024  CountFromType=Initial value  CountFrom=mp.DPRAM1_size-10  CountResetPort=off  CountLoadPort=on  CountEnbPort=on  CountDirPort=off  CountDataType=Unsigned  CountWordLen=mp.DPRAM1_address_size  CountFracLen=0  CountSampTime=1
      settings: SourceProductName=Simulink
  addr_B : Outport  VectorParamsAs1DForOutWhenUnconnected=off
  Frame_counter : Outport  Port=2  VectorParamsAs1DForOutWhenUnconnected=off
  FFT_Valid : Outport  Port=3  VectorParamsAs1DForOutWhenUnconnected=off
  wires:
  counter_B/1 -> addr_B/1
  start/1 -> counter_B/1, addr_B_gen_enable/1(start)
  addr_B_gen_enable/1(enable_B) -> Logical Operator1/1
  addr_B_gen_enable/2(Start_Address) -> counter_B/2
  enable/1 -> Logical Operator1/2
  addr_B_gen_enable/3(Frame_Index) -> Frame_counter/1
  Logical Operator1/1 -> counter_B/3, FFT_Valid/1

== system fft_filters/dataplane/FFT_Analysis_Synthesis_Left/Frequency_Domain_Processing/Apply_Complex_Gains/FFT_Filter_Coefficients ==
  select : Inport
  valid : Inport  Port=2
  FFT_ROM_Indexing : Subsystem
  Filter_ROM_Choice : Subsystem
  filter_gains : Outport
  wires:
  FFT_ROM_Indexing/1(ROM_index) -> Filter_ROM_Choice/2(Index)
  valid/1 -> FFT_ROM_Indexing/1(valid)
  select/1 -> Filter_ROM_Choice/1(select)
  Filter_ROM_Choice/1(filter_gains) -> filter_gains/1

== system fft_filters/dataplane/FFT_Analysis_Synthesis_Left/Synthesis/Overlap_and_Add/Hanning_ROM ==
  Index : Inport
  Bit Slice : hdlsllib/Logic and Bit Operations/Bit Slice  lidx=log2(mp.FFT_size) - 1  ridx=0
      settings: SourceProductName=Simulink  SourceProductBaseCode=SL
  Lookup Table : Lookup_n-D  NumberOfTableDimensions=1  BreakpointsForDimension1=[0:mp.FFT_size-1]  IndexSearchMethod=Evenly spaced points  Table=hanning(mp.FFT_size)  InterpMethod=Flat  ExtrapMethod=Clip  DiagnosticForOutOfRangeInput=Error  UseLastTableValue=on  OutDataTypeStr=fixdt(1,24,22)  RndMeth=Simplest  InputSameDT=on
  Unit Delay : UnitDelay  SampleTime=-1  HasFrameUpgradeWarning=on
  hanning_value : Outport  VectorParamsAs1DForOutWhenUnconnected=off
  wires:
  Unit Delay/1 -> hanning_value/1
  Index/1 -> Bit Slice/1
  Lookup Table/1 -> Unit Delay/1
  Bit Slice/1 -> Lookup Table/1

== system fft_filters/dataplane/FFT_Analysis_Synthesis_Right/Analysis/FFT Frame Buffering/FFT_pulse_gen ==
  note: Don't send out FFT frame start pulses
      | until circular buffer has filled.
  counter : Inport
  FFT_Frame_Pulse_Gen : Subsystem
  Wait_for_data_to_start : Subsystem
  FFT_start_pulse : Outport  VectorParamsAs1DForOutWhenUnconnected=off
  Enable_FFTs : Outport  Port=2  VectorParamsAs1DForOutWhenUnconnected=off
  wires:
  counter/1 -> FFT_Frame_Pulse_Gen/1("counter_value ")
  Wait_for_data_to_start/1(FFT_Frame_Start) -> FFT_start_pulse/1
  Wait_for_data_to_start/2(Enable_FFT_Frames) -> Enable_FFTs/1
  FFT_Frame_Pulse_Gen/1(Frame_Pulse) -> Wait_for_data_to_start/1(Frame_Pulse)

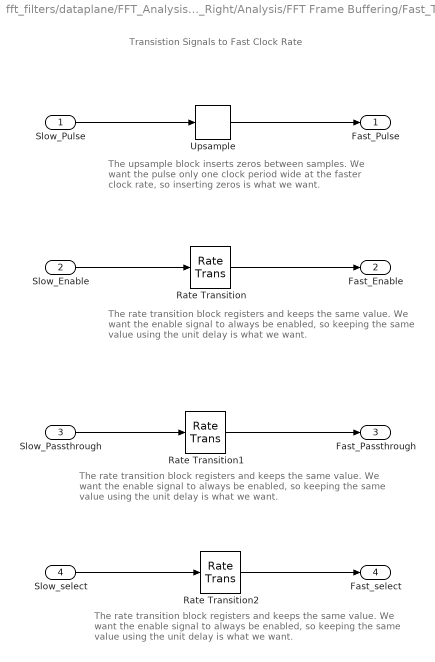
== system fft_filters/dataplane/FFT_Analysis_Synthesis_Right/Analysis/FFT Frame Buffering/Fast_Transition ==
  note: The upsample block inserts zeros between samples.
      | We want the pulse only one clock period wide at the
      | faster clock rate, so inserting zeros is what we want.
  note: Transistion Signals to Fast Clock Rate
  note: The rate transition block registers and keeps the same
      | value.  We want the enable signal to always be enabled,
      | so keeping the same value using the unit delay is what we want.
  note: The rate transition block registers and keeps the same
      | value.  We want the enable signal to always be enabled,
      | so keeping the same value using the unit delay is what we want.
  note: The rate transition block registers and keeps the same
      | value.  We want the enable signal to always be enabled,
      | so keeping the same value using the unit delay is what we want.
  Slow_Pulse : Inport
  Slow_Enable : Inport  Port=2
  Slow_Passthrough : Inport  Port=3
  Slow_select : Inport  Port=4
  Rate Transition : RateTransition  OutPortSampleTimeOpt=Multiple of input port sample time  OutPortSampleTimeMultiple=1/mp.SysRate_Upsample_Factor
  Rate Transition1 : RateTransition  OutPortSampleTimeOpt=Multiple of input port sample time  OutPortSampleTimeMultiple=1/mp.SysRate_Upsample_Factor
  Rate Transition2 : RateTransition  InitialCondition=3  OutPortSampleTimeOpt=Multiple of input port sample time  OutPortSampleTimeMultiple=1/mp.SysRate_Upsample_Factor
  Upsample : dspsigops/Upsample  N=mp.SysRate_Upsample_Factor  phase=0  RateOptions=Allow multirate processing  ic=0  mode=Unused parameter value
  Fast_Pulse : Outport
  Fast_Enable : Outport  Port=2
  Fast_Passthrough : Outport  Port=3
  Fast_select : Outport  Port=4
  wires:
  Slow_Pulse/1 -> Upsample/1
  Rate Transition/1 -> Fast_Enable/1
  Slow_Enable/1 -> Rate Transition/1
  Upsample/1 -> Fast_Pulse/1
  Slow_Passthrough/1 -> Rate Transition1/1
  Rate Transition1/1 -> Fast_Passthrough/1
  Slow_select/1 -> Rate Transition2/1
  Rate Transition2/1 -> Fast_select/1

== system fft_filters/dataplane/FFT_Analysis_Synthesis_Right/Analysis/FFT Frame Buffering/Hanning_ROM ==
  Index : Inport
  Bit Slice : hdlsllib/Logic and Bit Operations/Bit Slice  lidx=log2(mp.FFT_size) - 1  ridx=0
      settings: SourceProductName=Simulink  SourceProductBaseCode=SL
  Lookup Table : Lookup_n-D  NumberOfTableDimensions=1  BreakpointsForDimension1=[0:mp.FFT_size-1]  IndexSearchMethod=Evenly spaced points  Table=hanning(mp.FFT_size)  InterpMethod=Flat  ExtrapMethod=Clip  DiagnosticForOutOfRangeInput=Warning  UseLastTableValue=on  OutDataTypeStr=fixdt(1,24,23)  RndMeth=Simplest  InputSameDT=on
  Unit Delay : UnitDelay  SampleTime=-1  HasFrameUpgradeWarning=on
  hanning_value : Outport  VectorParamsAs1DForOutWhenUnconnected=off
  wires:
  Unit Delay/1 -> hanning_value/1
  Index/1 -> Bit Slice/1
  Lookup Table/1 -> Unit Delay/1
  Bit Slice/1 -> Lookup Table/1

== system fft_filters/dataplane/FFT_Analysis_Synthesis_Right/Analysis/FFT Frame Buffering/addr_A_offset ==
  note: Adding 1 to counter since the read pointer (addr_B) can catch the write pointer (addr_A)
      | if SysRate_Upsample_Factor is large enough and Simulink will throw an error.
      | It would be nice if the HDL Coder allowed a read-before-write option when
      | the addresses are identical, which some memories support.
  counter_A : Inport
  Add : Sum  OutDataTypeStr=fixdt(0,mp.DPRAM1_address_size,0)
  write_offset : Constant  OutDataTypeStr=fixdt(0,mp.DPRAM1_address_size,0)  SampleTime=mp.Ts
  addr_A : Outport  VectorParamsAs1DForOutWhenUnconnected=off
  wires:
  write_offset/1 -> Add/2
  Add/1 -> addr_A/1
  counter_A/1 -> Add/1

== system fft_filters/dataplane/FFT_Analysis_Synthesis_Right/Analysis/FFT Frame Buffering/addr_B_gen ==
  note: Counter values [0 FFT_size-1] that
      | is used to lookup the window values
      | being applied.
  note: Valid data is being streamed to the FFT Engine.
  note: Enable signal that indicates
      | there is data in the buffer
      | and FFTs can start.
  note: The start pulse sets the starting count to Start_Address
      |  and the counter counts from Start_Address to Start_Address + FFT_size - 1
      | which is the address sent to Port B of the dual port memory.
  start : Inport
  enable : Inport  Port=2
  Logical Operator1 : Logic  AllPortsSameDT=off  OutDataTypeStr=boolean
  addr_B_gen_enable : Subsystem
  counter_B : hdlsllib/Sources/HDL Counter  CountType=Free running  CountInit=mp.DPRAM1_size-10  CountStep=1  CountMax=1024  CountFromType=Initial value  CountFrom=mp.DPRAM1_size-10  CountResetPort=off  CountLoadPort=on  CountEnbPort=on  CountDirPort=off  CountDataType=Unsigned  CountWordLen=mp.DPRAM1_address_size  CountFracLen=0  CountSampTime=1
      settings: SourceProductName=Simulink
  addr_B : Outport  VectorParamsAs1DForOutWhenUnconnected=off
  Frame_counter : Outport  Port=2  VectorParamsAs1DForOutWhenUnconnected=off
  FFT_Valid : Outport  Port=3  VectorParamsAs1DForOutWhenUnconnected=off
  wires:
  counter_B/1 -> addr_B/1
  start/1 -> counter_B/1, addr_B_gen_enable/1(start)
  addr_B_gen_enable/1(enable_B) -> Logical Operator1/1
  addr_B_gen_enable/2(Start_Address) -> counter_B/2
  enable/1 -> Logical Operator1/2
  addr_B_gen_enable/3(Frame_Index) -> Frame_counter/1
  Logical Operator1/1 -> counter_B/3, FFT_Valid/1

== system fft_filters/dataplane/FFT_Analysis_Synthesis_Right/Frequency_Domain_Processing/Apply_Complex_Gains/FFT_Filter_Coefficients ==
  select : Inport
  valid : Inport  Port=2
  FFT_ROM_Indexing : Subsystem
  Filter_ROM_Choice : Subsystem
  filter_gains : Outport
  wires:
  FFT_ROM_Indexing/1(ROM_index) -> Filter_ROM_Choice/2(Index)
  valid/1 -> FFT_ROM_Indexing/1(valid)
  select/1 -> Filter_ROM_Choice/1(select)
  Filter_ROM_Choice/1(filter_gains) -> filter_gains/1

== system fft_filters/dataplane/FFT_Analysis_Synthesis_Right/Synthesis/Overlap_and_Add/Hanning_ROM ==
  Index : Inport
  Bit Slice : hdlsllib/Logic and Bit Operations/Bit Slice  lidx=log2(mp.FFT_size) - 1  ridx=0
      settings: SourceProductName=Simulink  SourceProductBaseCode=SL
  Lookup Table : Lookup_n-D  NumberOfTableDimensions=1  BreakpointsForDimension1=[0:mp.FFT_size-1]  IndexSearchMethod=Evenly spaced points  Table=hanning(mp.FFT_size)  InterpMethod=Flat  ExtrapMethod=Clip  DiagnosticForOutOfRangeInput=Error  UseLastTableValue=on  OutDataTypeStr=fixdt(1,24,22)  RndMeth=Simplest  InputSameDT=on
  Unit Delay : UnitDelay  SampleTime=-1  HasFrameUpgradeWarning=on
  hanning_value : Outport  VectorParamsAs1DForOutWhenUnconnected=off
  wires:
  Unit Delay/1 -> hanning_value/1
  Index/1 -> Bit Slice/1
  Lookup Table/1 -> Unit Delay/1
  Bit Slice/1 -> Lookup Table/1

== system fft_filters/dataplane/FFT_Analysis_Synthesis_Left/Analysis/FFT Frame Buffering/FFT_pulse_gen/FFT_Frame_Pulse_Gen ==
  note: Create a FFT frame pulse that happens every FFT_size/4 samples.
      | We do this by watching when an appropriate subset of the counter bits
      | become zero.
  "counter_value " : Inport
  Bit Slice : hdlsllib/Logic and Bit Operations/Bit Slice  lidx=log2(mp.FFT_frame_shift)-1  ridx=0
      settings: SourceProductName=Simulink  SourceProductBaseCode=SL
  Compare To Zero : simulink/Logic and Bit Operations/Compare To Zero  relop===  OutDataTypeStr=boolean
  Frame_Pulse : Outport  VectorParamsAs1DForOutWhenUnconnected=off
  wires:
  "counter_value "/1 -> Bit Slice/1
  Compare To Zero/1 -> Frame_Pulse/1
  Bit Slice/1 -> Compare To Zero/1

== system fft_filters/dataplane/FFT_Analysis_Synthesis_Left/Analysis/FFT Frame Buffering/FFT_pulse_gen/Wait_for_data_to_start ==
  note: Frame pulses don't start
      | coming through until
      | circular buffer has data.
  note: Counter starts a zero and counts number of frame pulses.
      | Counter remains enabled while frame count is less than 4.
      | As soon as the counter reaches 4, it is disabled, which then
      | enables the frame pulses to pass through.
  note: Frame_Pulse
      | will pass through
      | when enabled
  note: Number of Frames
      | to wait before starting
  note: Start performing FFTs after enough data has filled the circular buffer.
      | This is due to the fact that we don't want the read pointer (addr_B)
      | to catch up with the write pointer (addr_A) because if it does,
      | the DPRAM will throw an assertion error.
  note: Enable signal that that indicates
      | that FFTs can start since there is
      | data in the buffer.
  Frame_Pulse : Inport
  Bitwise Operator : simulink/Logic and Bit Operations/Bitwise Operator  logicop=NOT  UseBitMask=off  BitMask=bin2dec('11011001')  BitMaskRealWorld=Stored Integer
  Compare To Constant : simulink/Logic and Bit Operations/Compare To Constant  relop=<  const=4  OutDataTypeStr=boolean
  Initial_frame_count : hdlsllib/Sources/HDL Counter  CountType=Count limited  CountInit=0  CountStep=1  CountMax=4  CountFromType=Specify  CountFrom=0  CountResetPort=off  CountLoadPort=off  CountEnbPort=on  CountDirPort=off  CountDataType=Unsigned  CountWordLen=5  CountFracLen=0  CountSampTime=1
      settings: SourceProductName=Simulink
  Logical Operator : Logic  AllPortsSameDT=off  OutDataTypeStr=boolean
  Logical Operator1 : Logic  AllPortsSameDT=off  OutDataTypeStr=boolean
  FFT_Frame_Start : Outport  VectorParamsAs1DForOutWhenUnconnected=off
  Enable_FFT_Frames : Outport  Port=2  VectorParamsAs1DForOutWhenUnconnected=off
  wires:
  Logical Operator1/1 -> FFT_Frame_Start/1
  Frame_Pulse/1 -> Logical Operator/2, Logical Operator1/1
  Initial_frame_count/1 -> Compare To Constant/1
  Logical Operator/1 -> Initial_frame_count/1
  Compare To Constant/1 -> Bitwise Operator/1, Logical Operator/1
  Bitwise Operator/1 -> Enable_FFT_Frames/1, Logical Operator1/2
